simulink model "main"  (R2022a)
settings: Solver=FixedStepDiscrete  StartTime=0.0  StopTime=Inf  FixedStep=(50e-6)-(sim_en*4.995e-5)  RelTol=1e-3  EnableMultiTasking=on
model workspace (MAT data in the model file):
  Param : Simulink.Parameter (value not decoded)
  ac_ok : Simulink.Signal (value not decoded)
  ac_ok_120 : Simulink.Signal (value not decoded)
  bulk_voltage : Simulink.Signal (value not decoded)
  burstduty_integ_max : Simulink.Signal (value not decoded)
  burstduty_integ_min : Simulink.Signal (value not decoded)
  burstduty_ki : Simulink.Signal (value not decoded)
  burstduty_kp : Simulink.Signal (value not decoded)
  calib_ok : Simulink.Signal (value not decoded)
  can_addr1 : Simulink.Signal (value not decoded)
  can_addr2 : Simulink.Signal (value not decoded)
  can_addr3 : Simulink.Signal (value not decoded)
  can_addr4 : Simulink.Signal (value not decoded)
  can_data_rx : Simulink.Signal (value not decoded)
  can_data_tx : Simulink.Signal (value not decoded)
  can_timeout_120 : Simulink.Signal (value not decoded)
  chksum_scircv : Simulink.Signal (value not decoded)
  clllc_en_120 : Simulink.Signal (value not decoded)
  clllc_fault_120 : Simulink.Signal (value not decoded)
  clllc_ok_120 : Simulink.Signal (value not decoded)
  cmpss1h : Simulink.Signal (value not decoded)
  cmpss1l : Simulink.Signal (value not decoded)
  cmpss2h : Simulink.Signal (value not decoded)
  cmpss2l : Simulink.Signal (value not decoded)
  cmpss3h : Simulink.Signal (value not decoded)
  cmpss3l : Simulink.Signal (value not decoded)
  cmpss4h : Simulink.Signal (value not decoded)
  cmpss4l : Simulink.Signal (value not decoded)
  cmpss5h : Simulink.Signal (value not decoded)
  cmpss5l : Simulink.Signal (value not decoded)
  cmpss6h : Simulink.Signal (value not decoded)
  cmpss6l : Simulink.Signal (value not decoded)
  cmpss7h : Simulink.Signal (value not decoded)
  cmpss7l : Simulink.Signal (value not decoded)
  cmpss8h : Simulink.Signal (value not decoded)
  cmpss8l : Simulink.Signal (value not decoded)
  cnt_idle : Simulink.Signal (value not decoded)
  cnt_orps : Simulink.Signal (value not decoded)
  cnt_scircv : Simulink.Signal (value not decoded)
  cnt_scixmt : Simulink.Signal (value not decoded)
  cnt_scixmt_func : Simulink.Signal (value not decoded)
  cnt_temp_mux : Simulink.Signal (value not decoded)
  cnt_vdroop : Simulink.Signal (value not decoded)
  config_ok : Simulink.Signal (value not decoded)
  control_en : Simulink.Signal (value not decoded)
  cp_ready_120 : Simulink.Signal (value not decoded)
  d2d_en : Simulink.Signal (value not decoded)
  dchg_off : Simulink.Signal (value not decoded)
  debug_dacb : Simulink.Signal (value not decoded)
  debug_dacc : Simulink.Signal (value not decoded)
  debug_msg1 : Simulink.Signal (value not decoded)
  debug_msg2 : Simulink.Signal (value not decoded)
  debug_msg3 : Simulink.Signal (value not decoded)
  debug_msg4 : Simulink.Signal (value not decoded)
  debug_msg5 : Simulink.Signal (value not decoded)
  debug_msg6 : Simulink.Signal (value not decoded)
  dir_v2g : Simulink.Signal (value not decoded)
  eoss_llc1 : Simulink.Signal (value not decoded)
  eoss_llc2 : Simulink.Signal (value not decoded)
  eoss_orps : Simulink.Signal (value not decoded)
  fault_ocp : Simulink.Signal (value not decoded)
  fault_otp : Simulink.Signal (value not decoded)
  fault_ovp : Simulink.Signal (value not decoded)
  fut_en : Simulink.Signal (value not decoded)
  fwd_en_120 : Simulink.Signal (value not decoded)
  gain_llc1_sec_idc : Simulink.Signal (value not decoded)
  gain_llc1_temp_sr : Simulink.Signal (value not decoded)
  gain_llc2_sec_idc : Simulink.Signal (value not decoded)
  gain_vbat : Simulink.Signal (value not decoded)
  gain_vbulk : Simulink.Signal (value not decoded)
  gain_vout : Simulink.Signal (value not decoded)
  input_current_phasea : Simulink.Signal (value not decoded)
  input_current_phaseb : Simulink.Signal (value not decoded)
  input_current_phasec : Simulink.Signal (value not decoded)
  input_freq : Simulink.Signal (value not decoded)
  input_power : Simulink.Signal (value not decoded)
  input_voltage_phasea : Simulink.Signal (value not decoded)
  input_voltage_phaseb : Simulink.Signal (value not decoded)
  input_voltage_phasec : Simulink.Signal (value not decoded)
  ishare_arbiter : Simulink.Signal (value not decoded)
  ishare_thresh : Simulink.Signal (value not decoded)
  led_g : Simulink.Signal (value not decoded)
  led_r : Simulink.Signal (value not decoded)
  led_y : Simulink.Signal (value not decoded)
  llc1_burst_integ : Simulink.Signal (value not decoded)
  llc1_burstduty_buffer : Simulink.Signal (value not decoded)
  llc1_pfm_error : Simulink.Signal (value not decoded)
  llc1_pfm_integ : Simulink.Signal (value not decoded)
  llc1_pfm_prop : Simulink.Signal (value not decoded)
  llc1_pri_idc : Simulink.Signal (value not decoded)
  llc1_ps_buffer : Simulink.Signal (value not decoded)
  llc1_pspwm_error : Simulink.Signal (value not decoded)
  llc1_pspwm_integ : Simulink.Signal (value not decoded)
  llc1_pspwm_prop : Simulink.Signal (value not decoded)
  llc1_sec_idc : Simulink.Signal (value not decoded)
  llc1_temp_sr : Simulink.Signal (value not decoded)
  llc1_ts_tbctr_buffer : Simulink.Signal (value not decoded)
  llc2_burst_integ : Simulink.Signal (value not decoded)
  llc2_burstduty_buffer : Simulink.Signal (value not decoded)
  llc2_en : Simulink.Signal (value not decoded)
  llc2_en_buffer : Simulink.Signal (value not decoded)
  llc2_pfm_error : Simulink.Signal (value not decoded)
  llc2_pfm_integ : Simulink.Signal (value not decoded)
  llc2_pfm_prop : Simulink.Signal (value not decoded)
  llc2_pri_idc : Simulink.Signal (value not decoded)
  llc2_ps_buffer : Simulink.Signal (value not decoded)
  llc2_pspwm_error : Simulink.Signal (value not decoded)
  llc2_pspwm_integ : Simulink.Signal (value not decoded)
  llc2_pspwm_prop : Simulink.Signal (value not decoded)
  llc2_sec_idc : Simulink.Signal (value not decoded)
  llc2_temp_sr : Simulink.Signal (value not decoded)
  llc2_ts_tbctr_buffer : Simulink.Signal (value not decoded)
  loop_adcint : Simulink.Signal (value not decoded)
  loop_control : Simulink.Signal (value not decoded)
  loop_idle : Simulink.Signal (value not decoded)
  mid_bulk_voltage : Simulink.Signal (value not decoded)
  mode_120 : Simulink.Signal (value not decoded)
  mode_cc_cv : Simulink.Signal (value not decoded)
  myParam : mpt.Parameter (value not decoded)
  obc_ok_120 : Simulink.Signal (value not decoded)
  offset_llc1_sec_idc : Simulink.Signal (value not decoded)
  offset_llc1_temp_sr : Simulink.Signal (value not decoded)
  offset_llc2_sec_idc : Simulink.Signal (value not decoded)
  offset_vbat : Simulink.Signal (value not decoded)
  offset_vbulk : Simulink.Signal (value not decoded)
  offset_vout : Simulink.Signal (value not decoded)
  openloop_en : Simulink.Signal (value not decoded)
  openloop_fault_en : Simulink.Signal (value not decoded)
  ot_fault_120 : Simulink.Signal (value not decoded)
  pfc_en : Simulink.Signal (value not decoded)
  pfc_en_120 : Simulink.Signal (value not decoded)
  pfc_fw_revision : Simulink.Signal (value not decoded)
  pfc_fw_revision_bootloader : Simulink.Signal (value not decoded)
  pfc_fw_revision_debug : Simulink.Signal (value not decoded)
  pfc_ok : Simulink.Signal (value not decoded)
  pfc_ok_120 : Simulink.Signal (value not decoded)
  pfm_a0 : Simulink.Signal (value not decoded)
  pfm_a1 : Simulink.Signal (value not decoded)
  pfm_integ_max : Simulink.Signal (value not decoded)
  pfm_integ_min : Simulink.Signal (value not decoded)
  pfm_ki : Simulink.Signal (value not decoded)
  pfm_kp : Simulink.Signal (value not decoded)
  pri_fut_en : Simulink.Signal (value not decoded)
  pri_fut_en_buffer : Simulink.Signal (value not decoded)
  pri_halfbridge_en : Simulink.Signal (value not decoded)
  pri_halfbridge_en_buffer : Simulink.Signal (value not decoded)
  pspwm_integ_max : Simulink.Signal (value not decoded)
  pspwm_integ_min : Simulink.Signal (value not decoded)
  pspwm_ki : Simulink.Signal (value not decoded)
  pspwm_kp : Simulink.Signal (value not decoded)
  ref_idclink_max : Simulink.Signal (value not decoded)
  ref_iout : Simulink.Signal (value not decoded)
  ref_iout_calib : Simulink.Signal (value not decoded)
  ref_iout_llc1 : Simulink.Signal (value not decoded)
  ref_iout_llc1_calib : Simulink.Signal (value not decoded)
  ref_iout_llc2 : Simulink.Signal (value not decoded)
  ref_iout_llc2_calib : Simulink.Signal (value not decoded)
  ref_pout : Simulink.Signal (value not decoded)
  ref_ss_llc1 : Simulink.Signal (value not decoded)
  ref_ss_llc2 : Simulink.Signal (value not decoded)
  ref_ss_orps : Simulink.Signal (value not decoded)
  ref_vbat : Simulink.Signal (value not decoded)
  ref_vbat_calib : Simulink.Signal (value not decoded)
  ref_vbulk : Simulink.Signal (value not decoded)
  ref_vbulk_calib : Simulink.Signal (value not decoded)
  ref_vbulk_llc1_calib : Simulink.Signal (value not decoded)
  ref_vbulk_llc2_calib : Simulink.Signal (value not decoded)
  ref_vout : Simulink.Signal (value not decoded)
  ref_vout_calib : Simulink.Signal (value not decoded)
  relay_en : Simulink.Signal (value not decoded)
  reset_flag : Simulink.Signal (value not decoded)
  rev_en_120 : Simulink.Signal (value not decoded)
  runtime_control : Simulink.Signal (value not decoded)
  runtime_idle : Simulink.Signal (value not decoded)
  scircv_buffer : Simulink.Signal (value not decoded)
  scircv_buffer_tmp : Simulink.Signal (value not decoded)
  scircv_buffer_tmp_idx0 : Simulink.Signal (value not decoded)
  scircv_chksum : Simulink.Signal (value not decoded)
  scircv_chksum_ok : Simulink.Signal (value not decoded)
  scircv_parse_ok : Simulink.Signal (value not decoded)
  scixmt_buffer : Simulink.Signal (value not decoded)
  scixmt_chksum : Simulink.Signal (value not decoded)
  scixmt_func : Simulink.Signal (value not decoded)
  scixmt_word0_lsb : Simulink.Signal (value not decoded)
  scixmt_word0_msb : Simulink.Signal (value not decoded)
  scixmt_word1_lsb : Simulink.Signal (value not decoded)
  scixmt_word1_msb : Simulink.Signal (value not decoded)
  scixmt_word2_lsb : Simulink.Signal (value not decoded)
  scixmt_word2_msb : Simulink.Signal (value not decoded)
  scixmt_wr : Simulink.Signal (value not decoded)
  ss_step : Simulink.Signal (value not decoded)
  state_calib : Simulink.Signal (value not decoded)
  state_control : Simulink.Signal (value not decoded)
  state_hkeep : Simulink.Signal (value not decoded)
  status_cmpss : Simulink.Signal (value not decoded)
  status_control : Simulink.Signal (value not decoded)
  status_digin : Simulink.Signal (value not decoded)
  status_digout : Simulink.Signal (value not decoded)
  status_fault : Simulink.Signal (value not decoded)
  status_input : Simulink.Signal (value not decoded)
  status_pfc : Simulink.Signal (value not decoded)
  temp_inlet : Simulink.Signal (value not decoded)
  temp_llc1_fet_hs : Simulink.Signal (value not decoded)
  temp_llc2_fet_hs : Simulink.Signal (value not decoded)
  temp_mux : Simulink.Signal (value not decoded)
  temp_mux_s0 : Simulink.Signal (value not decoded)
  temp_mux_s1 : Simulink.Signal (value not decoded)
  temp_mux_s2 : Simulink.Signal (value not decoded)
  temp_outlet : Simulink.Signal (value not decoded)
  temp_pfc_fet_hsa : Simulink.Signal (value not decoded)
  temp_pfc_fet_hsb : Simulink.Signal (value not decoded)
  temp_pfc_fet_hsc : Simulink.Signal (value not decoded)
  temp_pfc_fet_lsa : Simulink.Signal (value not decoded)
  temp_pfc_fet_lsb : Simulink.Signal (value not decoded)
  temp_pfc_fet_lsc : Simulink.Signal (value not decoded)
  test_mode : Simulink.Signal (value not decoded)
  tfcv_cc : Simulink.Signal (value not decoded)
  tfcv_cc_llc2 : Simulink.Signal (value not decoded)
  tfcv_cv : Simulink.Signal (value not decoded)
  tfcv_sr_en : Simulink.Signal (value not decoded)
  tfv_assert_llc1_pri_idc : Simulink.Signal (value not decoded)
  tfv_assert_llc1_sec_idc : Simulink.Signal (value not decoded)
  tfv_assert_llc1_temp_sr : Simulink.Signal (value not decoded)
  tfv_assert_llc2_pri_idc : Simulink.Signal (value not decoded)
  tfv_assert_llc2_sec_idc : Simulink.Signal (value not decoded)
  tfv_assert_llc2_temp_sr : Simulink.Signal (value not decoded)
  tfv_assert_temp_outlet : Simulink.Signal (value not decoded)
  tfv_assert_vaux_uv : Simulink.Signal (value not decoded)
  tfv_assert_vbat : Simulink.Signal (value not decoded)
  tfv_assert_vbulk : Simulink.Signal (value not decoded)
  tfv_assert_vout : Simulink.Signal (value not decoded)
  tfv_cnt_tz : Simulink.Signal (value not decoded)
  tfv_deassert_llc1_pri_idc : Simulink.Signal (value not decoded)
  tfv_deassert_llc1_sec_idc : Simulink.Signal (value not decoded)
  tfv_deassert_llc1_temp_sr : Simulink.Signal (value not decoded)
  tfv_deassert_llc2_pri_idc : Simulink.Signal (value not decoded)
  tfv_deassert_llc2_sec_idc : Simulink.Signal (value not decoded)
  tfv_deassert_llc2_temp_sr : Simulink.Signal (value not decoded)
  tfv_deassert_temp_outlet : Simulink.Signal (value not decoded)
  tfv_deassert_vaux_uv : Simulink.Signal (value not decoded)
  tfv_deassert_vbat : Simulink.Signal (value not decoded)
  tfv_deassert_vbulk : Simulink.Signal (value not decoded)
  tfv_deassert_vout : Simulink.Signal (value not decoded)
  tfv_llc1_pri_idc : Simulink.Signal (value not decoded)
  tfv_llc1_sec_idc : Simulink.Signal (value not decoded)
  tfv_llc1_temp_sr : Simulink.Signal (value not decoded)
  tfv_llc2_pri_idc : Simulink.Signal (value not decoded)
  tfv_llc2_sec_idc : Simulink.Signal (value not decoded)
  tfv_llc2_temp_sr : Simulink.Signal (value not decoded)
  tfv_temp_outlet : Simulink.Signal (value not decoded)
  tfv_vaux_uv : Simulink.Signal (value not decoded)
  tfv_vbat : Simulink.Signal (value not decoded)
  tfv_vbulk : Simulink.Signal (value not decoded)
  tfv_vout : Simulink.Signal (value not decoded)
  timer_1ms : Simulink.Signal (value not decoded)
  tz : Simulink.Signal (value not decoded)
  valve_en : Simulink.Signal (value not decoded)
  vaux : Simulink.Signal (value not decoded)
  vbat : Simulink.Signal (value not decoded)
  vbulk : Simulink.Signal (value not decoded)
  vout : Simulink.Signal (value not decoded)
undefined symbols (not defined in the file or in its folder): CAN_O_INT, CANA_BASE, Down, GPTRIP1SEL, GPTRIP2SEL, TZ1, TZ2, Up
libraries: hdlsllib x159, simulink x94, c2802xlib x32, c2837xDlib x19, c2807xlib x16, c280xlib x13, canmsglib x8, idelinklib_common x2, c2000lib x1, c281xlib x1
(part 15 of 20)

== system main/Task_Manager/idle/idle_task/hkeep/tfv/hkeep/HKEEP.tfvTempOutlet ==
  input : Inport  OutDataTypeStr=uint16
  assert_lim : Inport  Port=2  OutDataTypeStr=uint16
  assert_vld : Inport  Port=3  OutDataTypeStr=uint16
  deassert_lim : Inport  Port=4  OutDataTypeStr=uint16
  deassert_vld : Inport  Port=5  OutDataTypeStr=uint16
  f : TriggerPort  TriggerType=function-call  VariantControl=(inherit)
      settings: CopyFcn=Stateflow.SLINSF.SimulinkMan.removeBlockPreDeleteFcn  PreDeleteFcn=Stateflow.SLINSF.SimulinkMan.unsafePredeleteFcn
  Constant1 : Constant  Value=[512, 683, 1024, 1365, 1638, 2048, 2559, 2730, 2925, 3150, 3276, 3561, 3723]  OutDataTypeStr=uint16
  Constant4 : Constant  Value=[0, 10, 20, 30, 40, 50, 60, 70, 80, 90, 100, 120, 140]  OutDataTypeStr=uint16
  Data Store Read1 : DataStoreRead  DataStoreName=timer_1ms  IndexOptions=Index vector (dialog)  Indices=1  OutputSizes=1
  Data Type Conversion : DataTypeConversion  OutDataTypeStr=boolean  SaturateOnIntegerOverflow=off  RndMeth=Floor
  Data Type Conversion1 : DataTypeConversion  OutDataTypeStr=uint16  SaturateOnIntegerOverflow=off  RndMeth=Floor
  Lookup Table Dynamic : simulink/Lookup Tables/Lookup Table Dynamic  LookUpMeth=Interpolation-Use End Values  OutDataType=fixdt('uint16')  OutScaling=[]  OutputDataTypeScalingMode=Specify via dialog  OutDataTypeStr=uint16  DoSatur=off
  MATLAB System : MATLABSystem  System=tfv_latch  SimulateUsing=Code generation
      mask Type: tfv_latch
      mask Display:
      | disp('tfv_latch');
      | port_label('input',1,'input');
      | port_label('input',2,'assert_lim');
      | port_label('input',3,'assert_vld');
      | port_label('input',4,'deassert_lim');
      | port_label('input',5,'deassert_vld');
      | port_label('input',6,'tmr');
      | port_label('output',1,'status');
  Rate Transition1 : RateTransition  Deterministic=off
  tfv_status : Outport  OutDataTypeStr=boolean  PortDimensions=1
  wires:
  Constant1/1 -> Lookup Table Dynamic/2
  Constant4/1 -> Lookup Table Dynamic/3
  Lookup Table Dynamic/1 -> Data Type Conversion1/1
  MATLAB System/1 -> Data Type Conversion/1
  deassert_vld/1 -> MATLAB System/5
  Data Store Read1/1 -> MATLAB System/6
  assert_vld/1 -> MATLAB System/3
  deassert_lim/1 -> MATLAB System/4
  assert_lim/1 -> MATLAB System/2
  Data Type Conversion1/1 -> MATLAB System/1
  input/1 -> Rate Transition1/1
  Data Type Conversion/1 -> tfv_status/1
  Rate Transition1/1 -> Lookup Table Dynamic/1

== system main/Task_Manager/idle/idle_task/hkeep/tfv/hkeep/HKEEP.tfvVauxUvp ==
  input : Inport  OutDataTypeStr=uint16
  assert_lim : Inport  Port=2  OutDataTypeStr=uint16
  assert_vld : Inport  Port=3  OutDataTypeStr=uint16
  deassert_lim : Inport  Port=4  OutDataTypeStr=uint16
  deassert_vld : Inport  Port=5  OutDataTypeStr=uint16
  f : TriggerPort  TriggerType=function-call  VariantControl=(inherit)
      settings: CopyFcn=Stateflow.SLINSF.SimulinkMan.removeBlockPreDeleteFcn  PreDeleteFcn=Stateflow.SLINSF.SimulinkMan.unsafePredeleteFcn
  Data Store Read1 : DataStoreRead  DataStoreName=timer_1ms  IndexOptions=Index vector (dialog)  Indices=1  OutputSizes=1
  Data Type Conversion : DataTypeConversion  OutDataTypeStr=boolean  SaturateOnIntegerOverflow=off  RndMeth=Floor
  MATLAB System : MATLABSystem  System=tfv_latch  SimulateUsing=Code generation
      mask Type: tfv_latch
      mask Display:
      | disp('tfv_latch');
      | port_label('input',1,'input');
      | port_label('input',2,'assert_lim');
      | port_label('input',3,'assert_vld');
      | port_label('input',4,'deassert_lim');
      | port_label('input',5,'deassert_vld');
      | port_label('input',6,'tmr');
      | port_label('output',1,'status');
  tfv_status : Outport  OutDataTypeStr=boolean  PortDimensions=1
  wires:
  MATLAB System/1 -> Data Type Conversion/1
  deassert_vld/1 -> MATLAB System/5
  Data Store Read1/1 -> MATLAB System/6
  assert_vld/1 -> MATLAB System/3
  deassert_lim/1 -> MATLAB System/4
  assert_lim/1 -> MATLAB System/2
  input/1 -> MATLAB System/1
  Data Type Conversion/1 -> tfv_status/1

== system main/Task_Manager/idle/idle_task/hkeep/tfv/hkeep/HKEEP.tfvVbat ==
  input : Inport  OutDataTypeStr=uint16  PortDimensions=1
  assert_lim : Inport  Port=2  OutDataTypeStr=uint16  PortDimensions=1
  assert_vld : Inport  Port=3  OutDataTypeStr=uint16  PortDimensions=1
  deassert_lim : Inport  Port=4  OutDataTypeStr=uint16  PortDimensions=1
  deassert_vld : Inport  Port=5  OutDataTypeStr=uint16  PortDimensions=1
  f : TriggerPort  TriggerType=function-call  VariantControl=(inherit)
      settings: CopyFcn=Stateflow.SLINSF.SimulinkMan.removeBlockPreDeleteFcn  PreDeleteFcn=Stateflow.SLINSF.SimulinkMan.unsafePredeleteFcn
  Data Store Read : DataStoreRead  DataStoreName=timer_1ms  IndexOptions=Index vector (dialog)  Indices=1  OutputSizes=1
  Data Type Conversion : DataTypeConversion  OutDataTypeStr=boolean  SaturateOnIntegerOverflow=off  RndMeth=Floor
  MATLAB System : MATLABSystem  System=tfv_latch  SimulateUsing=Code generation
      mask Type: tfv_latch
      mask Display:
      | disp('tfv_latch');
      | port_label('input',1,'input');
      | port_label('input',2,'assert_lim');
      | port_label('input',3,'assert_vld');
      | port_label('input',4,'deassert_lim');
      | port_label('input',5,'deassert_vld');
      | port_label('input',6,'tmr');
      | port_label('output',1,'status');
  tfv_status : Outport  OutDataTypeStr=boolean
  wires:
  MATLAB System/1 -> Data Type Conversion/1
  input/1 -> MATLAB System/1
  assert_lim/1 -> MATLAB System/2
  assert_vld/1 -> MATLAB System/3
  deassert_lim/1 -> MATLAB System/4
  deassert_vld/1 -> MATLAB System/5
  Data Store Read/1 -> MATLAB System/6
  Data Type Conversion/1 -> tfv_status/1

== system main/Task_Manager/idle/idle_task/hkeep/tfv/hkeep/HKEEP.tfvVbulk ==
  input : Inport  OutDataTypeStr=uint16  PortDimensions=1
  assert_lim : Inport  Port=2  OutDataTypeStr=uint16  PortDimensions=1
  assert_vld : Inport  Port=3  OutDataTypeStr=uint16  PortDimensions=1
  deassert_lim : Inport  Port=4  OutDataTypeStr=uint16  PortDimensions=1
  deassert_vld : Inport  Port=5  OutDataTypeStr=uint16  PortDimensions=1
  f : TriggerPort  TriggerType=function-call  VariantControl=(inherit)
      settings: CopyFcn=Stateflow.SLINSF.SimulinkMan.removeBlockPreDeleteFcn  PreDeleteFcn=Stateflow.SLINSF.SimulinkMan.unsafePredeleteFcn
  Data Store Read : DataStoreRead  DataStoreName=timer_1ms  IndexOptions=Index vector (dialog)  Indices=1  OutputSizes=1
  Data Type Conversion : DataTypeConversion  OutDataTypeStr=boolean  SaturateOnIntegerOverflow=off  RndMeth=Floor
  MATLAB System : MATLABSystem  System=tfv_latch  SimulateUsing=Code generation
      mask Type: tfv_latch
      mask Display:
      | disp('tfv_latch');
      | port_label('input',1,'input');
      | port_label('input',2,'assert_lim');
      | port_label('input',3,'assert_vld');
      | port_label('input',4,'deassert_lim');
      | port_label('input',5,'deassert_vld');
      | port_label('input',6,'tmr');
      | port_label('output',1,'status');
  tfv_status : Outport  OutDataTypeStr=boolean
  wires:
  MATLAB System/1 -> Data Type Conversion/1
  input/1 -> MATLAB System/1
  assert_lim/1 -> MATLAB System/2
  assert_vld/1 -> MATLAB System/3
  deassert_lim/1 -> MATLAB System/4
  deassert_vld/1 -> MATLAB System/5
  Data Store Read/1 -> MATLAB System/6
  Data Type Conversion/1 -> tfv_status/1

== system main/Task_Manager/idle/idle_task/hkeep/tfv/hkeep/HKEEP.tfvVout ==
  input : Inport  OutDataTypeStr=uint16  PortDimensions=1
  assert_lim : Inport  Port=2  OutDataTypeStr=uint16  PortDimensions=1
  assert_vld : Inport  Port=3  OutDataTypeStr=uint16  PortDimensions=1
  deassert_lim : Inport  Port=4  OutDataTypeStr=uint16  PortDimensions=1
  deassert_vld : Inport  Port=5  OutDataTypeStr=uint16  PortDimensions=1
  f : TriggerPort  TriggerType=function-call  VariantControl=(inherit)
      settings: CopyFcn=Stateflow.SLINSF.SimulinkMan.removeBlockPreDeleteFcn  PreDeleteFcn=Stateflow.SLINSF.SimulinkMan.unsafePredeleteFcn
  Data Store Read : DataStoreRead  DataStoreName=timer_1ms  IndexOptions=Index vector (dialog)  Indices=1  OutputSizes=1
  Data Type Conversion : DataTypeConversion  OutDataTypeStr=boolean  SaturateOnIntegerOverflow=off  RndMeth=Floor
  tfv : MATLABSystem  System=tfv_latch  SimulateUsing=Code generation
      mask Type: tfv_latch
      mask Display:
      | disp('tfv_latch');
      | port_label('input',1,'input');
      | port_label('input',2,'assert_lim');
      | port_label('input',3,'assert_vld');
      | port_label('input',4,'deassert_lim');
      | port_label('input',5,'deassert_vld');
      | port_label('input',6,'tmr');
      | port_label('output',1,'status');
  tfv_status : Outport  OutDataTypeStr=boolean
  wires:
  tfv/1 -> Data Type Conversion/1
  input/1 -> tfv/1
  assert_lim/1 -> tfv/2
  assert_vld/1 -> tfv/3
  deassert_lim/1 -> tfv/4
  deassert_vld/1 -> tfv/5
  Data Store Read/1 -> tfv/6
  Data Type Conversion/1 -> tfv_status/1

== system main/Task_Manager/idle/idle_task/hkeep/tz/System Outputs ==

== system main/Task_Manager/idle/idle_task/hkeep/tz/System Outputs1 ==

== system main/Task_Manager/idle/idle_task/hkeep/tz/System Outputs2 ==

== system main/Task_Manager/idle/idle_task/hkeep/tz/System Outputs3 ==

== system main/Task_Manager/idle/idle_task/hkeep/tz/System Outputs4 ==

== system main/Task_Manager/idle/idle_task/status/init/digin//digout_variant_subsystem ==
  note: 1) Add Subsystem or Model blocks as valid variant choices.
      | 2) You cannot connect blocks at this level. At simulation, connectivity is automatically
      | determined, based on the active variant and port name matching.
  sim_digin : Inport
  codgen : Subsystem  VariantControl=sim_en==0
  sim : Subsystem  VariantControl=sim_en==1
  sim_digout : Outport

== system main/Task_Manager/idle/idle_task/status/update_CAN_msg1/OBC_CTRL_MSG_100 ==
  Cast To Double : DataTypeConversion  OutDataTypeStr=uint16  SaturateOnIntegerOverflow=off  RndMeth=Floor
  Cast To Double1 : DataTypeConversion  OutDataTypeStr=uint16  SaturateOnIntegerOverflow=off  RndMeth=Floor
  Data Store Read1 : DataStoreRead  DataStoreName=f32VoutTarget  IndexOptions=Index vector (dialog)  Indices=1  OutputSizes=1
  Data Store Read2 : DataStoreRead  DataStoreName=f32IoutTarget  IndexOptions=Index vector (dialog)  Indices=1  OutputSizes=1
  Data Store Read4 : DataStoreRead  DataStoreName=u8ModeCmd  IndexOptions=Index vector (dialog)  Indices=1  OutputSizes=1
  Data Store Write : DataStoreWrite  DataStoreName=ref_vbat  IndexOptions=Index vector (dialog)  Indices=1  OutputSizes=1
  Data Store Write1 : DataStoreWrite  DataStoreName=ref_iout_llc1  IndexOptions=Index vector (dialog)  Indices=1  OutputSizes=1
  G2V_Forward_ON_A2 : Subsystem
  Sleep_A0 : Subsystem
  Stand-by_A1 : Subsystem
  Switch Case : SwitchCase  CaseConditions={160,161,162,163,164,165}
  Test_mode_ON_AND_FWD_A4 : Subsystem
  Test_mode_ON_AND_REV_A5 : Subsystem
  V2G_Reverse_ON_A3 : Subsystem
  wires:
  Data Store Read4/1 -> Switch Case/1
  Switch Case/3 -> G2V_Forward_ON_A2/Action
  Switch Case/4 -> V2G_Reverse_ON_A3/Action
  Switch Case/1 -> Sleep_A0/Action
  Switch Case/2 -> Stand-by_A1/Action
  Switch Case/5 -> Test_mode_ON_AND_FWD_A4/Action
  Data Store Read1/1 -> Cast To Double/1
  Cast To Double/1 -> Data Store Write/1
  Switch Case/6 -> Test_mode_ON_AND_REV_A5/Action
  Cast To Double1/1 -> Data Store Write1/1
  Data Store Read2/1 -> Cast To Double1/1

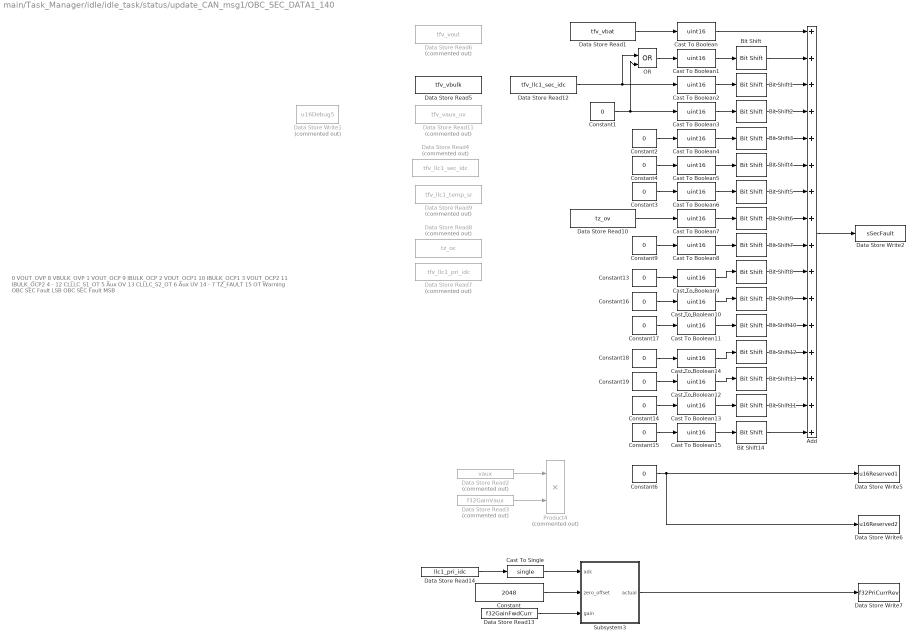
== system main/Task_Manager/idle/idle_task/status/update_CAN_msg1/OBC_SEC_DATA1_140 ==
  note: 0 VOUT_OVP 8 VBULK_OVP
      | 1 VOUT_OCP 9 IBULK_OCP
      | 2 VOUT_OCP1 10 IBULK_OCP1
      | 3 VOUT_OCP2 11 IBULK_OCP2
      | 4 - 12 CLLLC_S1_OT
      | 5 Aux OV 13 CLLLC_S2_OT
      | 6 Aux UV 14 -
      | 7 TZ_FAULT 15 OT Warning
      | OBC SEC Fault LSB OBC SEC Fault MSB
  Add : Sum  Inputs=++++++++++++++++
  Bit Shift : hdlsllib/Logic and Bit Operations/Bit Shift  mode=Shift Left Logical  N=1
  Bit Shift1 : hdlsllib/Logic and Bit Operations/Bit Shift  mode=Shift Left Logical  N=2
  Bit Shift10 : hdlsllib/Logic and Bit Operations/Bit Shift  mode=Shift Left Logical  N=11
  Bit Shift11 : hdlsllib/Logic and Bit Operations/Bit Shift  mode=Shift Left Logical  N=14
  Bit Shift12 : hdlsllib/Logic and Bit Operations/Bit Shift  mode=Shift Left Logical  N=12
  Bit Shift13 : hdlsllib/Logic and Bit Operations/Bit Shift  mode=Shift Left Logical  N=13
  Bit Shift14 : hdlsllib/Logic and Bit Operations/Bit Shift  mode=Shift Left Logical  N=15
  Bit Shift2 : hdlsllib/Logic and Bit Operations/Bit Shift  mode=Shift Left Logical  N=3
  Bit Shift3 : hdlsllib/Logic and Bit Operations/Bit Shift  mode=Shift Left Logical  N=4
  Bit Shift4 : hdlsllib/Logic and Bit Operations/Bit Shift  mode=Shift Left Logical  N=5
  Bit Shift5 : hdlsllib/Logic and Bit Operations/Bit Shift  mode=Shift Left Logical  N=6
  Bit Shift6 : hdlsllib/Logic and Bit Operations/Bit Shift  mode=Shift Left Logical  N=7
  Bit Shift7 : hdlsllib/Logic and Bit Operations/Bit Shift  mode=Shift Left Logical  N=8
  Bit Shift8 : hdlsllib/Logic and Bit Operations/Bit Shift  mode=Shift Left Logical  N=9
  Bit Shift9 : hdlsllib/Logic and Bit Operations/Bit Shift  mode=Shift Left Logical  N=10
  Cast To Boolean{,1..15} (16 alike) : DataTypeConversion  OutDataTypeStr=uint16  SaturateOnIntegerOverflow=off  RndMeth=Floor
  Cast To Single : DataTypeConversion  OutDataTypeStr=single  SaturateOnIntegerOverflow=off  RndMeth=Floor
  Constant : Constant  Value=2048  OutDataTypeStr=single
  Constant{1..4,6,9,13..19} (13 alike) : Constant  Value=0  OutDataTypeStr=uint16
  Data Store Read1 : DataStoreRead  DataStoreName=tfv_vbat  IndexOptions=Index vector (dialog)  Indices=1  OutputSizes=1
  Data Store Read10 : DataStoreRead  DataStoreName=tz_ov  IndexOptions=Index vector (dialog)  Indices=1  OutputSizes=1
  Data Store Read11 : DataStoreRead  Commented=on  DataStoreName=tfv_vaux_uv  IndexOptions=Index vector (dialog)  Indices=1  OutputSizes=1
  Data Store Read12 : DataStoreRead  DataStoreName=tfv_llc1_sec_idc  IndexOptions=Index vector (dialog)  Indices=1  OutputSizes=1
  Data Store Read13 : DataStoreRead  DataStoreName=f32GainFwdCurr  IndexOptions=Index vector (dialog)  Indices=1  OutputSizes=1
  Data Store Read14 : DataStoreRead  DataStoreName=llc1_pri_idc  IndexOptions=Index vector (dialog)  Indices=1  OutputSizes=1
  Data Store Read2 : DataStoreRead  Commented=on  DataStoreName=vaux  IndexOptions=Index vector (dialog)  Indices=1  OutputSizes=1
  Data Store Read3 : DataStoreRead  Commented=on  DataStoreName=f32GainVaux  IndexOptions=Index vector (dialog)  Indices=1  OutputSizes=1
  Data Store Read4 : DataStoreRead  Commented=on  DataStoreName=tfv_llc1_sec_idc  IndexOptions=Index vector (dialog)  Indices=1  OutputSizes=1
  Data Store Read5 : DataStoreRead  DataStoreName=tfv_vbulk  IndexOptions=Index vector (dialog)  Indices=1  OutputSizes=1
  Data Store Read6 : DataStoreRead  Commented=on  DataStoreName=tfv_vout  IndexOptions=Index vector (dialog)  Indices=1  OutputSizes=1
  Data Store Read7 : DataStoreRead  Commented=on  DataStoreName=tfv_llc1_pri_idc  IndexOptions=Index vector (dialog)  Indices=1  OutputSizes=1
  Data Store Read8 : DataStoreRead  Commented=on  DataStoreName=tz_oc  IndexOptions=Index vector (dialog)  Indices=1  OutputSizes=1
  Data Store Read9 : DataStoreRead  Commented=on  DataStoreName=tfv_llc1_temp_sr  IndexOptions=Index vector (dialog)  Indices=1  OutputSizes=1
  Data Store Write1 : DataStoreWrite  Commented=on  DataStoreName=u16Debug5  IndexOptions=Index vector (dialog)  Indices=1  OutputSizes=1
  Data Store Write2 : DataStoreWrite  DataStoreName=sSecFault  IndexOptions=Index vector (dialog)  Indices=1  OutputSizes=1
  Data Store Write5 : DataStoreWrite  DataStoreName=u16Reserved1  IndexOptions=Index vector (dialog)  Indices=1  OutputSizes=1
  Data Store Write6 : DataStoreWrite  DataStoreName=u16Reserved2  IndexOptions=Index vector (dialog)  Indices=1  OutputSizes=1
  Data Store Write7 : DataStoreWrite  DataStoreName=f32PriCurrRev  IndexOptions=Index vector (dialog)  Indices=1  OutputSizes=1
  OR : Logic  Operator=OR  IconShape=distinctive  AllPortsSameDT=off  OutDataTypeStr=boolean
  Product4 : Product  Commented=on  OutDataTypeStr=uint16
  Subsystem3 : Subsystem
  wires:
  Subsystem3/1(actual) -> Data Store Write7/1
  Cast To Boolean8/1 -> Bit Shift7/1
  Cast To Boolean11/1 -> Bit Shift10/1
  Bit Shift10/1 -> Add/12
  Bit Shift9/1 -> Add/11
  Cast To Boolean10/1 -> Bit Shift9/1
  Bit Shift7/1 -> Add/9
  Bit Shift1/1 -> Add/3
  Cast To Boolean4/1 -> Bit Shift3/1
  Bit Shift8/1 -> Add/10
  Bit Shift6/1 -> Add/8
  Bit Shift/1 -> Add/2
  OR/1 -> Cast To Boolean1/1
  Cast To Boolean5/1 -> Bit Shift4/1
  Bit Shift4/1 -> Add/6
  Bit Shift5/1 -> Add/7
  Bit Shift2/1 -> Add/4
  Cast To Boolean6/1 -> Bit Shift5/1
  Cast To Boolean/1 -> Add/1
  Add/1 -> Data Store Write2/1
  Cast To Boolean3/1 -> Bit Shift2/1
  Bit Shift3/1 -> Add/5
  Cast To Boolean2/1 -> Bit Shift1/1
  Cast To Boolean7/1 -> Bit Shift6/1
  Constant1/1 -> OR/2, Cast To Boolean3/1
  Data Store Read1/1 -> Cast To Boolean/1
  Constant4/1 -> Cast To Boolean5/1
  Cast To Boolean9/1 -> Bit Shift8/1
  Cast To Boolean1/1 -> Bit Shift/1
  Cast To Boolean14/1 -> Bit Shift12/1
  Bit Shift12/1 -> Add/13
  Cast To Boolean12/1 -> Bit Shift13/1
  Bit Shift13/1 -> Add/14
  Bit Shift11/1 -> Add/15
  Cast To Boolean13/1 -> Bit Shift11/1
  Cast To Boolean15/1 -> Bit Shift14/1
  Bit Shift14/1 -> Add/16
  Constant14/1 -> Cast To Boolean13/1
  Constant13/1 -> Cast To Boolean9/1
  Constant18/1 -> Cast To Boolean14/1
  Constant15/1 -> Cast To Boolean15/1
  Constant16/1 -> Cast To Boolean10/1
  Constant19/1 -> Cast To Boolean12/1
  Constant17/1 -> Cast To Boolean11/1
  Data Store Read3/1 -> Product4/2
  Data Store Read2/1 -> Product4/1
  Constant6/1 -> Data Store Write6/1, Data Store Write5/1
  Data Store Read10/1 -> Cast To Boolean7/1
  Constant9/1 -> Cast To Boolean8/1
  Constant2/1 -> Cast To Boolean4/1
  Constant3/1 -> Cast To Boolean6/1
  Data Store Read12/1 -> OR/1, Cast To Boolean2/1
  Cast To Single/1 -> Subsystem3/1(adc)
  Constant/1 -> Subsystem3/2(zero_offset)
  Data Store Read14/1 -> Cast To Single/1
  Data Store Read13/1 -> Subsystem3/3(gain)

== system main/Task_Manager/idle/idle_task/status/update_CAN_msg1/OBC_SEC_DATA2_141 ==
  Cast To Double1 : DataTypeConversion  OutDataTypeStr=single  SaturateOnIntegerOverflow=off  RndMeth=Floor
  Cast To Double2 : DataTypeConversion  OutDataTypeStr=single  SaturateOnIntegerOverflow=off  RndMeth=Floor
  Constant10 : Constant  Value=0  OutDataTypeStr=single
  Constant12 : Constant  Value=0  OutDataTypeStr=single
  Data Store Read1 : DataStoreRead  DataStoreName=f32PriCurrRev  IndexOptions=Index vector (dialog)  Indices=1  OutputSizes=1
  Data Store Read10 : DataStoreRead  DataStoreName=f32Iout  IndexOptions=Index vector (dialog)  Indices=1  OutputSizes=1
  Data Store Write10 : DataStoreWrite  DataStoreName=f32PriCurrRev1  IndexOptions=Index vector (dialog)  Indices=1  OutputSizes=1
  Data Store Write11 : DataStoreWrite  DataStoreName=f32PriCurrRev2  IndexOptions=Index vector (dialog)  Indices=1  OutputSizes=1
  Data Store Write8 : DataStoreWrite  DataStoreName=f32Iout1  IndexOptions=Index vector (dialog)  Indices=1  OutputSizes=1
  Data Store Write9 : DataStoreWrite  DataStoreName=f32Iout2  IndexOptions=Index vector (dialog)  Indices=1  OutputSizes=1
  wires:
  Cast To Double2/1 -> Data Store Write10/1
  Constant10/1 -> Data Store Write9/1
  Constant12/1 -> Data Store Write11/1
  Cast To Double1/1 -> Data Store Write8/1
  Data Store Read10/1 -> Cast To Double1/1
  Data Store Read1/1 -> Cast To Double2/1

== system main/Task_Manager/idle/idle_task/status/update_CAN_msg1/OBC_SEC_DATA3_142 ==
  Constant{1..3,17} (4 alike) : Constant  Value=0  OutDataTypeStr=uint8
  Constant19 : Constant  Value=0  OutDataTypeStr=single
  Constant20 : Constant  Value=0  OutDataTypeStr=single
  Data Store Write14 : DataStoreWrite  DataStoreName=u8TclllcS3  IndexOptions=Index vector (dialog)  Indices=1  OutputSizes=1
  Data Store Write15 : DataStoreWrite  DataStoreName=u8TclllcS1  IndexOptions=Index vector (dialog)  Indices=1  OutputSizes=1
  Data Store Write16 : DataStoreWrite  DataStoreName=u8TclllcS2  IndexOptions=Index vector (dialog)  Indices=1  OutputSizes=1
  Data Store Write17 : DataStoreWrite  DataStoreName=u8TclllcS4  IndexOptions=Index vector (dialog)  Indices=1  OutputSizes=1
  Data Store Write18 : DataStoreWrite  DataStoreName=f32IshareErr  IndexOptions=Index vector (dialog)  Indices=1  OutputSizes=1
  Data Store Write19 : DataStoreWrite  DataStoreName=f32IshareAdj  IndexOptions=Index vector (dialog)  Indices=1  OutputSizes=1
  wires:
  Constant17/1 -> Data Store Write17/1
  Constant19/1 -> Data Store Write18/1
  Constant3/1 -> Data Store Write16/1
  Constant20/1 -> Data Store Write19/1
  Constant1/1 -> Data Store Write14/1
  Constant2/1 -> Data Store Write15/1

== system main/Task_Manager/idle/idle_task/status/update_CAN_msg1/OBC_SEC_DATA4_143 ==
  note: sSecCtrlState
      | 0 CTRL Mode 0-Burst, 1 - PSPWM, 2 - PFM
      | 1
      | 2 Ctrl Mode - 0-CC, 1-CV
      | 3 SR_Enabled
      | 4 Ishare Enabled
      | 5 -
      | 6 -
      | 7 -
  Add : Sum  Inputs=+++++++
  Bit Shift1 : hdlsllib/Logic and Bit Operations/Bit Shift  mode=Shift Left Logical  N=2
  Bit Shift2 : hdlsllib/Logic and Bit Operations/Bit Shift  mode=Shift Left Logical  N=3
  Bit Shift3 : hdlsllib/Logic and Bit Operations/Bit Shift  mode=Shift Left Logical  N=4
  Bit Shift4 : hdlsllib/Logic and Bit Operations/Bit Shift  mode=Shift Left Logical  N=5
  Bit Shift5 : hdlsllib/Logic and Bit Operations/Bit Shift  mode=Shift Left Logical  N=6
  Bit Shift6 : hdlsllib/Logic and Bit Operations/Bit Shift  mode=Shift Left Logical  N=7
  Cast To Boolean{1..7} (7 alike) : DataTypeConversion  OutDataTypeStr=uint16  SaturateOnIntegerOverflow=off  RndMeth=Floor
  Cast To Single : DataTypeConversion  OutDataTypeStr=uint8  SaturateOnIntegerOverflow=off  RndMeth=Floor
  Cast To Single1 : DataTypeConversion  OutDataTypeStr=uint8  SaturateOnIntegerOverflow=off  RndMeth=Floor
  Cast To Single2 : DataTypeConversion  OutDataTypeStr=single  SaturateOnIntegerOverflow=off  RndMeth=Floor
  Cast To Single3 : DataTypeConversion  OutDataTypeStr=uint8  SaturateOnIntegerOverflow=off  RndMeth=Floor
  Constant{1..5} (5 alike) : Constant  Value=0  OutDataTypeStr=uint16
  Constant21 : Constant  Value=0  OutDataTypeStr=uint8
  Constant23 : Constant  Value=0  OutDataTypeStr=uint8
  Constant25 : Constant  Value=0  OutDataTypeStr=single
  Data Store Read : DataStoreRead  DataStoreName=llc1_ts_tbctr  IndexOptions=Index vector (dialog)  Indices=1  OutputSizes=1
  Data Store Read1 : DataStoreRead  DataStoreName=llc1_ps  IndexOptions=Index vector (dialog)  Indices=1  OutputSizes=1
  Data Store Read2 : DataStoreRead  DataStoreName=llc1_burstduty  IndexOptions=Index vector (dialog)  Indices=1  OutputSizes=1
  Data Store Read3 : DataStoreRead  DataStoreName=mode  IndexOptions=Index vector (dialog)  Indices=1  OutputSizes=1
  Data Store Read5 : DataStoreRead  DataStoreName=mode_cc_cv  IndexOptions=Index vector (dialog)  Indices=1  OutputSizes=1
  Data Store Write12 : DataStoreWrite  DataStoreName=sSecCtrlState  IndexOptions=Index vector (dialog)  Indices=1  OutputSizes=1
  Data Store Write13 : DataStoreWrite  DataStoreName=u8BurstDty1  IndexOptions=Index vector (dialog)  Indices=1  OutputSizes=1
  Data Store Write20 : DataStoreWrite  DataStoreName=u8BurstDty2  IndexOptions=Index vector (dialog)  Indices=1  OutputSizes=1
  Data Store Write21 : DataStoreWrite  DataStoreName=u8PhaseShift1  IndexOptions=Index vector (dialog)  Indices=1  OutputSizes=1
  Data Store Write22 : DataStoreWrite  DataStoreName=u8PhaseShift2  IndexOptions=Index vector (dialog)  Indices=1  OutputSizes=1
  Data Store Write23 : DataStoreWrite  DataStoreName=f32Period1  IndexOptions=Index vector (dialog)  Indices=1  OutputSizes=1
  Data Store Write24 : DataStoreWrite  DataStoreName=f32Period2  IndexOptions=Index vector (dialog)  Indices=1  OutputSizes=1
  Subsystem : Subsystem  Commented=on
  wires:
  Constant23/1 -> Data Store Write22/1
  Constant25/1 -> Data Store Write24/1
  Constant21/1 -> Data Store Write20/1
  Data Store Read1/1 -> Cast To Single1/1
  Cast To Single/1 -> Data Store Write13/1
  Data Store Read2/1 -> Cast To Single/1
  Cast To Single1/1 -> Data Store Write21/1
  Data Store Read/1 -> Cast To Single2/1
  Cast To Single2/1 -> Data Store Write23/1
  Constant3/1 -> Cast To Boolean6/1
  Bit Shift3/1 -> Add/4
  Constant5/1 -> Cast To Boolean7/1
  Constant4/1 -> Cast To Boolean5/1
  Constant2/1 -> Cast To Boolean4/1
  Cast To Boolean5/1 -> Bit Shift4/1
  Cast To Boolean7/1 -> Bit Shift6/1
  Constant1/1 -> Cast To Boolean3/1
  Bit Shift4/1 -> Add/5
  Cast To Boolean2/1 -> Bit Shift1/1
  Cast To Boolean6/1 -> Bit Shift5/1
  Cast To Boolean3/1 -> Bit Shift2/1
  Bit Shift6/1 -> Add/7
  Bit Shift5/1 -> Add/6
  Bit Shift1/1 -> Add/2
  Cast To Boolean4/1 -> Bit Shift3/1
  Bit Shift2/1 -> Add/3
  Add/1 -> Cast To Single3/1
  Data Store Read5/1 -> Cast To Boolean2/1
  Data Store Read3/1 -> Cast To Boolean1/1
  Cast To Single3/1 -> Data Store Write12/1
  Cast To Boolean1/1 -> Add/1

== system main/Task_Manager/idle/idle_task/status/update_CAN_msg1/OBC_SEC_REQ_DEBUG_DATA_146_147 ==
  note: MSG ID 0x146
  note: MSG ID 0x147
  Cast To Single{,1..5} (6 alike) : DataTypeConversion  OutDataTypeStr=uint16  SaturateOnIntegerOverflow=off  RndMeth=Floor
  Constant : Constant  Value=1000
  DAC1 : c2837xDlib/DAC  channel=C  saturate=off
      settings: SourceProductBaseCode=TIC2000
  Data Store Read : DataStoreRead  DataStoreName=vbat  IndexOptions=Index vector (dialog)  Indices=1  OutputSizes=1
  Data Store Read1 : DataStoreRead  Commented=on  DataStoreName=f32Vout  IndexOptions=Index vector (dialog)  Indices=1  OutputSizes=1
  Data Store Read2 : DataStoreRead  Commented=on  DataStoreName=vaux  IndexOptions=Index vector (dialog)  Indices=1  OutputSizes=1
  Data Store Read3 : DataStoreRead  Commented=on  DataStoreName=f32GainVaux  IndexOptions=Index vector (dialog)  Indices=1  OutputSizes=1
  Data Store Read4 : DataStoreRead  DataStoreName=precharge_count  IndexOptions=Index vector (dialog)  Indices=1  OutputSizes=1
  Data Store Read5 : DataStoreRead  DataStoreName=eoss_llc1  IndexOptions=Index vector (dialog)  Indices=1  OutputSizes=1
  Data Store Read6 : DataStoreRead  DataStoreName=llc1_sec_idc  IndexOptions=Index vector (dialog)  Indices=1  OutputSizes=1
  Data Store Read7 : DataStoreRead  DataStoreName=ref_iout_llc1_calib  IndexOptions=Index vector (dialog)  Indices=1  OutputSizes=1
  Data Store Read8 : DataStoreRead  DataStoreName=ref_vbat_calib  IndexOptions=Index vector (dialog)  Indices=1  OutputSizes=1
  Data Store Write1 : DataStoreWrite  DataStoreName=u16Debug5  IndexOptions=Index vector (dialog)  Indices=1  OutputSizes=1
  Data Store Write25 : DataStoreWrite  DataStoreName=u16Debug1  IndexOptions=Index vector (dialog)  Indices=1  OutputSizes=1
  Data Store Write26 : DataStoreWrite  DataStoreName=u16Debug0  IndexOptions=Index vector (dialog)  Indices=1  OutputSizes=1
  Data Store Write27 : DataStoreWrite  DataStoreName=u16Debug2  IndexOptions=Index vector (dialog)  Indices=1  OutputSizes=1
  Data Store Write28 : DataStoreWrite  DataStoreName=u16Debug4  IndexOptions=Index vector (dialog)  Indices=1  OutputSizes=1
  Data Store Write29 : DataStoreWrite  DataStoreName=u16Debug3  IndexOptions=Index vector (dialog)  Indices=1  OutputSizes=1
  Product1 : Product  OutDataTypeStr=uint16
  Product4 : Product  Commented=on  OutDataTypeStr=uint16
  wires:
  Data Store Read4/1 -> Cast To Single2/1
  Data Store Read5/1 -> Product1/2, Cast To Single3/1
  Data Store Read8/1 -> Cast To Single1/1
  Data Store Read/1 -> Cast To Single/1
  Cast To Single/1 -> Data Store Write25/1
  Data Store Read3/1 -> Product4/2
  Data Store Read2/1 -> Product4/1
  Cast To Single1/1 -> Data Store Write27/1
  Cast To Single2/1 -> Data Store Write26/1
  Cast To Single3/1 -> Data Store Write29/1
  Data Store Read6/1 -> Cast To Single4/1
  Cast To Single4/1 -> Data Store Write28/1
  Data Store Read7/1 -> Cast To Single5/1
  Product1/1 -> DAC1/1
  Constant/1 -> Product1/1
  Cast To Single5/1 -> Data Store Write1/1

== system main/Task_Manager/idle/idle_task/status/update_CAN_msg1/OBC_SEC_STAT_MSG_120 ==
  Cast To Double4 : DataTypeConversion  OutDataTypeStr=single  SaturateOnIntegerOverflow=off  RndMeth=Floor
  Cast To Double6 : DataTypeConversion  OutDataTypeStr=single  SaturateOnIntegerOverflow=off  RndMeth=Floor
  Cast To Single : DataTypeConversion  OutDataTypeStr=single  SaturateOnIntegerOverflow=off  RndMeth=Floor
  Constant : Constant  Value=2006  OutDataTypeStr=single
  Constant1 : Constant  Value=0.0397  OutDataTypeStr=single
  Data Store Read1 : DataStoreRead  DataStoreName=llc1_sec_idc  IndexOptions=Index vector (dialog)  Indices=1  OutputSizes=1
  Data Store Read11 : DataStoreRead  DataStoreName=f32GainVBulk  IndexOptions=Index vector (dialog)  Indices=1  OutputSizes=1
  Data Store Read12 : DataStoreRead  DataStoreName=vbat  IndexOptions=Index vector (dialog)  Indices=1  OutputSizes=1
  Data Store Read3 : DataStoreRead  DataStoreName=f32GainVbat  IndexOptions=Index vector (dialog)  Indices=1  OutputSizes=1
  Data Store Read8 : DataStoreRead  DataStoreName=vbulk  IndexOptions=Index vector (dialog)  Indices=1  OutputSizes=1
  Data Store Write1 : DataStoreWrite  DataStoreName=f32Iout  IndexOptions=Index vector (dialog)  Indices=1  OutputSizes=1
  Data Store Write4 : DataStoreWrite  DataStoreName=f32Vout  IndexOptions=Index vector (dialog)  Indices=1  OutputSizes=1
  Data Store Write6 : DataStoreWrite  DataStoreName=f32Vbulk  IndexOptions=Index vector (dialog)  Indices=1  OutputSizes=1
  Product4 : Product  OutDataTypeStr=single
  Product5 : Product  OutDataTypeStr=single
  Subsystem : Subsystem
  Subsystem3 : Subsystem
  wires:
  Data Store Read12/1 -> Product5/1
  Data Store Read3/1 -> Product5/2
  Product5/1 -> Cast To Double4/1
  Product4/1 -> Cast To Double6/1
  Data Store Read11/1 -> Product4/2
  Cast To Double6/1 -> Data Store Write6/1
  Cast To Double4/1 -> Data Store Write4/1
  Data Store Read8/1 -> Product4/1
  Constant1/1 -> Subsystem3/3(gain)
  Subsystem3/1(actual) -> Data Store Write1/1
  Constant/1 -> Subsystem3/2(zero_offset)
  Data Store Read1/1 -> Cast To Single/1
  Cast To Single/1 -> Subsystem3/1(adc)

== system main/Task_Manager/idle/idle_task/uartx/parse/System Outputs3 ==

== system main/Task_Manager/init/codegen/init/outputxbar/System Initialize1 ==

== system main/Task_Manager/init/codegen/init/outputxbar/System Initialize2 ==

== system main/Task_Manager/init/codegen/init/outputxbar/System Initialize3 ==

== system main/Task_Manager/init/codegen/init/outputxbar/System Initialize4 ==

== system main/Task_Manager/init/codegen/init/outputxbar/System Initialize5 ==

== system main/Task_Manager/init/codegen/init/outputxbar/System Initialize6 ==

== system main/Task_Manager/init/codegen/init/pwmsync/System Initialize ==

== system main/Task_Manager/init/codegen/init/pwmsync/System Initialize1 ==

== system main/Task_Manager/init/codegen/init/pwmsync/System Initialize2 ==
